simulink library "drives_lib"  (Simulink 6.0)
settings: Solver=ode45  SolverMode=SingleTasking  StartTime=0.0  StopTime=10.0  RelTol=1e-3
libraries: simulink_extras x2, simulink3 x1
settings Model: LastModifiedBy=studadm
settings OptimizationCC: BooleanDataType=off
settings DebuggingCC: SolverPrmCheckMsg=none
settings HardwareCC: TargetUnknown=on

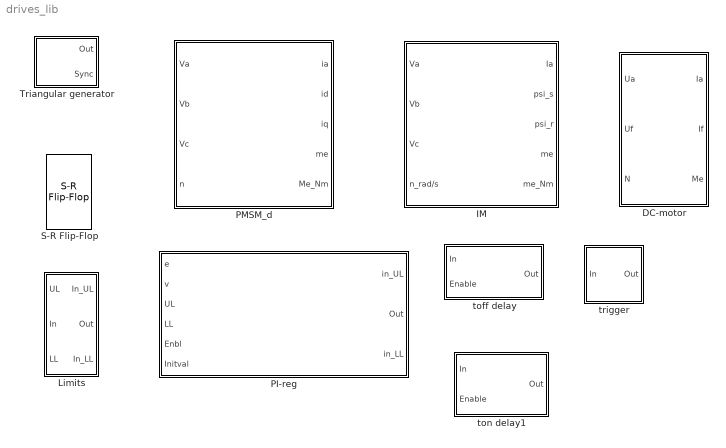
== system drives_lib ==
  DC-motor : Subsystem  mask{U_aN=400, I_aN=2.5, U_fN=310, I_fN=7, n_ref=1000, Ra_ref=160, MN=8, Ra=0.5, La=0.005, Tf=0.1}
      mask prompts: U_aN "U_an, anker merkespenning [V]"; I_aN "I_aN, anker merkestrøm [A]"; U_fN "U_fn, felt merkespenning [V]"; I_fN "I_fn, felt merkestrøm [A]"; n_ref "n_ref, merketurtall [o/min]"; Ra_ref "Ra_ref, basismotstand [ohm]"; MN "MN, merkemoment [Nm]"; Ra "Ra, ankermotstand [ohm]"; La "La, anker induktans [H]"; Tf "Tf, tidskonstant i feltkrets [sek]"
      mask help: DC-motor med skalering til pu-verdier
      mask Display:
      | text(0.25,0.7,'Likestrøm')
      | text(0.25,0.6,'maskin')
  IM : Subsystem  mask{Sn=10000, Un=400, fn=50, p=2, rs=0.04, rr=0.03, xh=2.273, xs=2.375, xr=2.385}
      mask prompts: Sn "Sn, merkeeffekt [VA]"; Un "Un, merke linjespenning [V]"; fn "fn, merkefrevens [Hz]"; p "p, antall polpar"; rs "rs, statorresistans [p.u]"; rr "rr, rotorresistans [p.u]"; xh "xh, magnetiseringsresistans [p.u]"; xs "xs, statorreaktans"; xr "xr, rotorreaktans"
      mask help:
      | Denne modulen er en asynkronmotormodul (kortslutningsmotor).
      | Modulen er basert paa invers-gamma transformasjonen.
      | Tilstandsvariable er stator strom i alfa og beta akse, og
      | rotor fluks i alfa og beta akse.
      mask Display:
      | text(0.20,0.9,'Induction machine')
      | 
      | 
      | plot([0.2500    0.2600    0.2700    0.2900    0.3100    0.3300    0.3600    0.3900    0.4200    0.4600    0.5000    0.5400    0.5800    0.6100    0.6400    0.6700    0.6900    0.7100    0.7300    0.7400    0.7500], [0.6000    0.6700    0.6980    0.7356    0.7625    0.7833    0.8071    0.8245    0.8369    0.8468    0.8500    0.8468    0.8369    0.8245    0.8071    0.7833    0.7625    0.7356    0.6980    0.6700    0.6000])
      | plot([0.2500    0.2600    0.2700    0.2900    0.3100    0.3300    0.3600    0.3900    0.4200    0.4600    0.5000    0.5400    0.5800    0.6100    0.6400    0.6700    0.6900    0.7100    0.7300    0.7400    0.7500], [0.6000    0.5300    0.5020    0.4644    0.4375    0.4167    0.3929    0.3755    0.3631    0.3532    0.3500    0.3532    0.3631    0.3755    0.3929    0.4167    0.4375    0.4644    0.5020    0.5300    0.6000])
      | 
      | plot([0.3250    0.3320    0.3390    0.3530    0.3670    0.3810    0.4020    0.4230    0.4440    0.4720    0.5000    0.5280    0.5560    0.5770    0.5980    0.6190    0.6330    0.6470    0.6610    0.6680    0.6750], [0.6000    0.6490    0.6686    0.6950    0.7137    0.7283    0.7450    0.7571    0.7658    0.7727    0.7750    0.7727    0.7658    0.7571    0.7450    0.7283    0.7137    0.6950    0.6686    0.6490    0.6000])
      | plot([0.3250    0.3320    0.3390    0.3530    0.3670    0.3810    0.4020    0.4230    0.4440    0.4720    0.5000    0.5280    0.5560    0.5770    0.5980    0.6190    0.6330    0.6470    0.6610    0.6680    0.6750], [0.6000    0.5510    0.5314    0.5050    0.4863    0.4717    0.4550    0.4429    0.4342    0.4273    0.4250    0.4273    0.4342    0.4429    0.4550    0.4717    0.4863    0.5050    0.5314    0.5510    0.6000])
      | 
      | plot([0.4 0.4 0.44 0.44 0.4],   [0.55 0.65 0.65 0.55 0.55])
      | plot([0.56 0.56 0.6 0.6 0.56], [0.55 0.65 0.65 0.55 0.55])
      | plot([0.45 0.55 0.55 0.45 0.45], [0.5 0.5 0.53 0.53 0.5])
      | plot([0.45 0.55 0.55 0.45 0.45], [0.7 0.7 0.67 0.67 0.7])
      | 
      | plot([0.495 0.505 0.755 0.745 0.495], [0.595 0.605 0.355 0.345 0.595])
  Limits : Subsystem
      mask Display:
      | plot([0.3 0.5 0.7 0.3], [0.1 0.3  0.1 0.1])
      | plot([0.3 0.5 0.7 0.3], [0.9 0.7  0.9 0.9])
  PI-reg : Subsystem  mask{Kp=0.3234, Kv=0, Ti=12e-3}
      mask Display:
      | plot([0.2 0.8], [0.1 0.1])
      | plot([0.2 0.2], [0.1 0.9])
      | plot([0.75 0.8 0.75], [0.15 0.1 0.05])
      | plot([0.175 0.2 0.225], [0.79 0.9 0.79])
      | 
      | plot([0.2 0.75], [0.3 0.7])
  PMSM_d : Subsystem  mask{Sn=3000, p=4, Un=230, fn=50, xd=0.5, xq=1.0, xls=0.06, xlkd=0.15, xlkq=0.15, rs=0.02, rkd=0.05, rkq=0.1, im=1.0}
      mask prompts: Sn "Sn, merkeeffekt [VA]"; p "p, antall polpar"; Un "Un, merkespenning (line-line rms) [V]"; fn "fn, merkefrekvens [Hz]"; xd "xd, reaktans i d-akse [p.u]"; xq "xq, reaktans i q-akse [p.u]"; xls "x_ls, lekkreaktans i stator [p.u]"; xlkd "x_lkd, lekkreaktans i dempevikl. d-akse [p.u]"; xlkq "x_lkq, lekkreaktans i dempevikl. q-akse [p.u]"; rs "rs, pr. fase statorresistans [p.u]"; rkd "r_kd, resistans i dempevikl. d-akse [p.u]"; rkq "r_kq, resistans i dempevikl. q-akse [p.u]"; im "i_m, ekv. magnetiseringsstrøm [p.u]"
      mask help:
      | dq-transformert modell av en permanentmagnetisert
      | synkronmotor (PMSM) med dempeviklinger.
      mask Display:
      | text(0.15,0.9,'PM Synch. Machine')
      | text(0.2,0.25,'w/damperwindings')
      | 
      | plot([0.2500    0.2600    0.2700    0.2900    0.3100    0.3300    0.3600    0.3900    0.4200    0.4600    0.5000    0.5400    0.5800    0.6100    0.6400    0.6700    0.6900    0.7100    0.7300    0.7400    0.7500], [0.6000    0.6700    0.6980    0.7356    0.7625    0.7833    0.8071    0.8245    0.8369    0.8468    0.8500    0.8468    0.8369    0.8245    0.8071    0.7833    0.7625    0.7356    0.6980    0.6700    0.6000])
      | plot([0.2500    0.2600    0.2700    0.2900    0.3100    0.3300    0.3600    0.3900    0.4200    0.4600    0.5000    0.5400    0.5800    0.6100    0.6400    0.6700    0.6900    0.7100    0.7300    0.7400    0.7500], [0.6000    0.5300    0.5020    0.4644    0.4375    0.4167    0.3929    0.3755    0.3631    0.3532    0.3500    0.3532    0.3631    0.3755    0.3929    0.4167    0.4375    0.4644    0.5020    0.5300    0.6000])
      | 
      | plot([0.3250    0.3320    0.3390    0.3530    0.3670    0.3810    0.4020    0.4230    0.4440    0.4720    0.5000    0.5280    0.5560    0.5770    0.5980    0.6190    0.6330    0.6470    0.6610    0.6680    0.6750], [0.6000    0.6490    0.6686    0.6950    0.7137    0.7283    0.7450    0.7571    0.7658    0.7727    0.7750    0.7727    0.7658    0.7571    0.7450    0.7283    0.7137    0.6950    0.6686    0.6490    0.6000])
      | plot([0.3250    0.3320    0.3390    0.3530    0.3670    0.3810    0.4020    0.4230    0.4440    0.4720    0.5000    0.5280    0.5560    0.5770    0.5980    0.6190    0.6330    0.6470    0.6610    0.6680    0.6750], [0.6000    0.5510    0.5314    0.5050    0.4863    0.4717    0.4550    0.4429    0.4342    0.4273    0.4250    0.4273    0.4342    0.4429    0.4550    0.4717    0.4863    0.5050    0.5314    0.5510    0.6000])
      | 
      | plot([0.4 0.4 0.44 0.44 0.4],   [0.55 0.65 0.65 0.55 0.55])
      | plot([0.56 0.56 0.6 0.6 0.56], [0.55 0.65 0.65 0.55 0.55])
      | plot([0.45 0.55 0.55 0.45 0.45], [0.5 0.5 0.53 0.53 0.5])
      | plot([0.45 0.55 0.55 0.45 0.45], [0.7 0.7 0.67 0.67 0.7])
      | 
      | plot([0.495 0.505 0.755 0.745 0.495], [0.595 0.605 0.355 0.345 0.595])
  S-R Flip-Flop : simulink_extras/Flip Flops/S-R Flip-Flop  initial_condition=0
  Triangular generator : Subsystem  mask(Triangular wave generator){ftri=1000, A=1, O=0}
      mask prompts: ftri "Frequency [Hz]"; A "Amplitude"; O "Offset"
      mask help:
      | Outputs a triangular waveform between -Amplitude and
      | +Amplitude with the set frequency and an optional offset.
      | The sync signal goes high at +Ampl. and low at -Ampl.
      mask Display: plot([0 0.1 0.2 0.3 0.4 0.5 0.6 ],[0 1 0 1 0 1 0])
  toff delay : Subsystem  mask{td=0.05}
      mask prompts: td "tidsforsinkelse td [s]:"
      mask help:
      | Når inngangen går høy, går utgangen momentant høy. Når inngangen går lav, går utgangen
      | lav etter en tidsforsinkelse td. Prosessen overstyres av Enable.
      mask Display:
      | plot([0.3 0.4 0.4 0.6 0.6 0.7 ],[0.7  0.7 1 1 0.7 0.7])
      | plot([0.3 0.4 0.4 0.65 0.65 0.7 ],[0.3  0.3 0.6 0.6 0.3 0.3])
  ton delay1 : Subsystem  AncestorBlock=eea_lib/ton delay  mask{td=0.8}
      mask prompts: td "tidsforsinkelse td [s]:"
      mask help:
      | Når inngangen går høy, går utgangen høy etter en tidsforsinkelse td. Når inngangen går lav, går utgangen
      | lavt momentant. Prosessen overstyres av Enable.
      mask Display:
      | plot([0.3 0.4 0.4 0.6 0.6 0.7 ],[0.7  0.7 1 1 0.7 0.7])
      | plot([0.3 0.45 0.45 0.6 0.6 0.7 ],[0.3  0.3 0.6 0.6 0.3 0.3])
  trigger : Subsystem  mask{ton=}
      mask prompts: ton "Påtid, ton [s]:"
      mask help:
      | Når inngangen går høy,
      |  går utgangen høy i en tid lik ton.
      mask Display:
      | plot([0.1 0.15 0.15 0.20 0.20 0.4  0.45 0.45 0.5 0.5 0.6],[0.7  0.7 1 1 0.7 0.7 0.7 1 1 0.7 0.7])
      | plot([0.1 0.15 0.15 0.35 0.35 0.4 0.45 0.45 0.6 ],[0.3 0.3 0.6 0.6 0.3 0.3 0.3 0.6 0.6])
      | plot([0.15 0.17],[0.48 0.48])
      | plot([0.33 0.35],[0.48 0.48])
      | text(0.21,0.5,'ton')

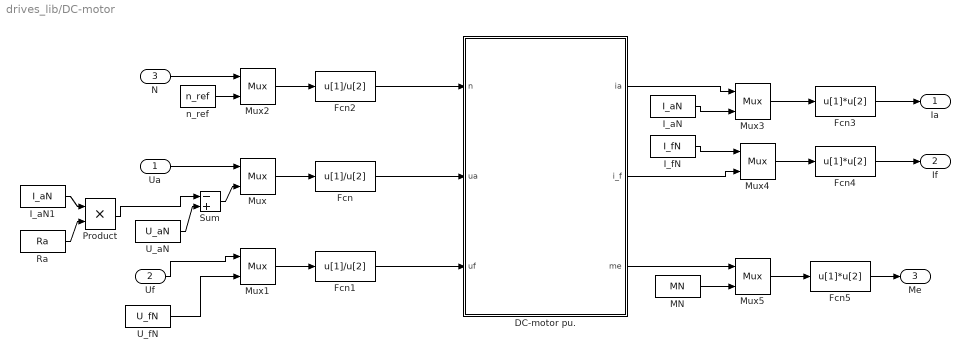
== system drives_lib/DC-motor ==
  Ua : Inport  Port=1  LatchInput=off
  Uf : Inport  Port=2  LatchInput=off
  N : Inport  Port=3  LatchInput=off
  DC-motor pu. : Subsystem
  Fcn : Fcn  Expr=u[1]/u[2]
  Fcn1 : Fcn  Expr=u[1]/u[2]
  Fcn2 : Fcn  Expr=u[1]/u[2]
  Fcn3 : Fcn  Expr=u[1]*u[2]
  Fcn4 : Fcn  Expr=u[1]*u[2]
  Fcn5 : Fcn  Expr=u[1]*u[2]
  I_aN : Constant  Value=I_aN
  I_aN1 : Constant  Value=I_aN
  I_fN : Constant  Value=I_fN
  MN : Constant  Value=MN
  Mux{,1..5} (6 alike) : Mux  Inputs=2
  Product : Product  SaturateOnIntegerOverflow=on  RndMeth=Zero  InputSameDT=on
  Ra : Constant  Value=Ra
  Sum : Sum  Inputs=-+  SaturateOnIntegerOverflow=on  InputSameDT=on
  U_aN : Constant  Value=U_aN
  U_fN : Constant  Value=U_fN
  n_ref : Constant  Value=n_ref
  Ia : Outport  InitialOutput=0
  If : Outport  Port=2  InitialOutput=0
  Me : Outport  Port=3  InitialOutput=0
  wires:
  N/1 -> Mux2/1
  Mux2/1 -> Fcn2/1
  n_ref/1 -> Mux2/2
  Fcn2/1 -> DC-motor pu./1(n)
  Ua/1 -> Mux/1
  Mux/1 -> Fcn/1
  Fcn/1 -> DC-motor pu./2(ua)
  Uf/1 -> Mux1/1
  Mux1/1 -> Fcn1/1
  Fcn1/1 -> DC-motor pu./3(uf)
  DC-motor pu./2(i_f) -> Mux4/2
  DC-motor pu./1(ia) -> Mux3/1
  I_aN/1 -> Mux3/2
  Mux3/1 -> Fcn3/1
  Mux4/1 -> Fcn4/1
  Fcn3/1 -> Ia/1
  Fcn4/1 -> If/1
  MN/1 -> Mux5/2
  Mux5/1 -> Fcn5/1
  Fcn5/1 -> Me/1
  DC-motor pu./3(me) -> Mux5/1
  Sum/1 -> Mux/2
  U_aN/1 -> Sum/2
  Product/1 -> Sum/1
  I_aN1/1 -> Product/1
  Ra/1 -> Product/2
  U_fN/1 -> Mux1/2
  I_fN/1 -> Mux4/1

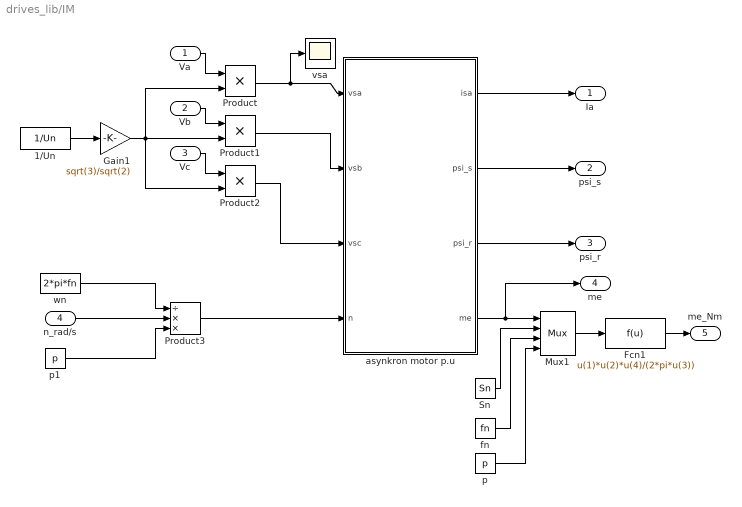
== system drives_lib/IM ==
  Va : Inport  Port=1  LatchInput=off
  Vb : Inport  Port=2  LatchInput=off
  Vc : Inport  Port=3  LatchInput=off
  n_rad/s : Inport  Port=4  LatchInput=off
  1/Un : Constant  Value=1/Un
  Fcn1 : Fcn  Expr=u(1)*u(2)*u(4)/(2*pi*u(3))
  Gain1 : Gain  Gain=sqrt(3)/sqrt(2)  SaturateOnIntegerOverflow=on
  Mux1 : Mux
  Product : Product  SaturateOnIntegerOverflow=on  RndMeth=Zero  InputSameDT=on
  Product1 : Product  SaturateOnIntegerOverflow=on  RndMeth=Zero  InputSameDT=on
  Product2 : Product  SaturateOnIntegerOverflow=on  RndMeth=Zero  InputSameDT=on
  Product3 : Product  Inputs=/**  SaturateOnIntegerOverflow=on  RndMeth=Zero  InputSameDT=on
  Sn : Constant  Value=Sn
  asynkron motor p.u : Subsystem
  fn : Constant  Value=fn
  p : Constant  Value=p
  p1 : Constant  Value=p
  vsa : Scope
      settings: TickLabels=on  YMin=-25  YMax=15  DataFormat=Array
  wn : Constant  Value=2*pi*fn
  Ia : Outport  InitialOutput=0
  psi_s : Outport  Port=2  InitialOutput=0
  psi_r : Outport  Port=3  InitialOutput=0
  me : Outport  Port=4  InitialOutput=0
  me_Nm : Outport  Port=5  InitialOutput=0
  wires:
  asynkron motor p.u/3(psi_r) -> psi_r/1
  asynkron motor p.u/2("psi_s ") -> psi_s/1
  Vc/1 -> Product2/1
  asynkron motor p.u/1(isa) -> Ia/1
  Vb/1 -> Product1/1
  Va/1 -> Product/1
  Product2/1 -> asynkron motor p.u/3(vsc)
  Product1/1 -> asynkron motor p.u/2(vsb)
  Fcn1/1 -> me_Nm/1
  Sn/1 -> Mux1/2
  Mux1/1 -> Fcn1/1
  fn/1 -> Mux1/3
  p/1 -> Mux1/4
  asynkron motor p.u/4(me) -> me/1, Mux1/1
  Gain1/1 -> Product1/2, Product/2, Product2/2
  1/Un/1 -> Gain1/1
  Product/1 -> asynkron motor p.u/1(vsa), vsa/1
  n_rad/s/1 -> Product3/2
  Product3/1 -> asynkron motor p.u/4(n)
  p1/1 -> Product3/3
  wn/1 -> Product3/1

== system drives_lib/Limits ==
  UL : Inport  Port=1  LatchInput=off
  In : Inport  Port=2  LatchInput=off
  LL : Inport  Port=3  LatchInput=off
  LL-test : MinMax  Function=max  Inputs=2  SaturateOnIntegerOverflow=on  InputSameDT=on
  Sum : Sum  Inputs=|-+  SaturateOnIntegerOverflow=on  InputSameDT=on
  Sum1 : Sum  Inputs=-+|  SaturateOnIntegerOverflow=on  InputSameDT=on
  UL-test : MinMax  Inputs=2  SaturateOnIntegerOverflow=on  InputSameDT=on
  in LL : Relay  OnSwitchValue=0  OffSwitchValue=-eps
  in UL : Relay  OnSwitchValue=0  OffSwitchValue=-eps
  In_UL : Outport
  Out : Outport  Port=2
  In_LL : Outport  Port=3
  wires:
  UL-test/1 -> LL-test/1, Sum/2
  Sum1/1 -> in LL/1
  LL-test/1 -> Sum1/1, Out/1
  UL/1 -> UL-test/1, Sum/1
  LL/1 -> LL-test/2, Sum1/2
  In/1 -> UL-test/2
  in LL/1 -> In_LL/1
  Sum/1 -> in UL/1
  in UL/1 -> In_UL/1

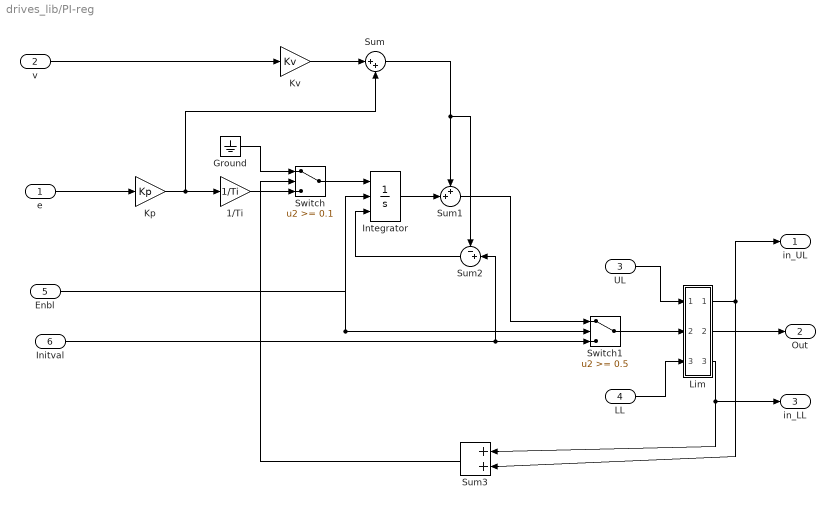
== system drives_lib/PI-reg ==
  e : Inport  Port=1  LatchInput=off
  v : Inport  Port=2  LatchInput=off
  UL : Inport  Port=3  LatchInput=off
  LL : Inport  Port=4  LatchInput=off
  Enbl : Inport  Port=5  LatchInput=off
  Initval : Inport  Port=6  LatchInput=off
  1/Ti : Gain  Gain=1/Ti  SaturateOnIntegerOverflow=on
  Ground : Ground
  Integrator : Integrator  ExternalReset=rising  InitialConditionSource=external
  Kp : Gain  Gain=Kp  SaturateOnIntegerOverflow=on
  Kv : Gain  Gain=Kv  SaturateOnIntegerOverflow=on
  Lim : Subsystem
      mask Display:
      | plot([0.3 0.5 0.7 0.3], [0.1 0.3  0.1 0.1])
      | plot([0.3 0.5 0.7 0.3], [0.9 0.7  0.9 0.9])
  Sum : Sum  Inputs=|++  SaturateOnIntegerOverflow=on  InputSameDT=on
  Sum1 : Sum  Inputs=++|  SaturateOnIntegerOverflow=on  InputSameDT=on
  Sum2 : Sum  Orientation=left  Inputs=-+|  SaturateOnIntegerOverflow=on  InputSameDT=on
  Sum3 : Sum  Orientation=left  Inputs=++|  SaturateOnIntegerOverflow=on  InputSameDT=on
  Switch : Switch  Threshold=0.1  SaturateOnIntegerOverflow=on  InputSameDT=on
  Switch1 : Switch  Threshold=0.5  SaturateOnIntegerOverflow=on  InputSameDT=on
  in_UL : Outport
  Out : Outport  Port=2
  in_LL : Outport  Port=3
  wires:
  Lim/3(In_LL) -> in_LL/1, Sum3/1
  Lim/2(Out) -> Out/1
  Lim/1(In_UL) -> in_UL/1, Sum3/2
  LL/1 -> Lim/3(LL)
  e/1 -> Kp/1
  UL/1 -> Lim/1(UL)
  v/1 -> Kv/1
  Sum3/1 -> Switch/2
  Sum2/1 -> Integrator/3
  Initval/1 -> Sum2/2, Switch1/3
  Sum/1 -> Sum2/1, Sum1/1
  Enbl/1 -> Integrator/2, Switch1/2
  Sum1/1 -> Switch1/1
  Integrator/1 -> Sum1/2
  Kp/1 -> Sum/2, 1/Ti/1
  Ground/1 -> Switch/1
  1/Ti/1 -> Switch/3
  Switch/1 -> Integrator/1
  Switch1/1 -> Lim/2(In)
  Kv/1 -> Sum/1

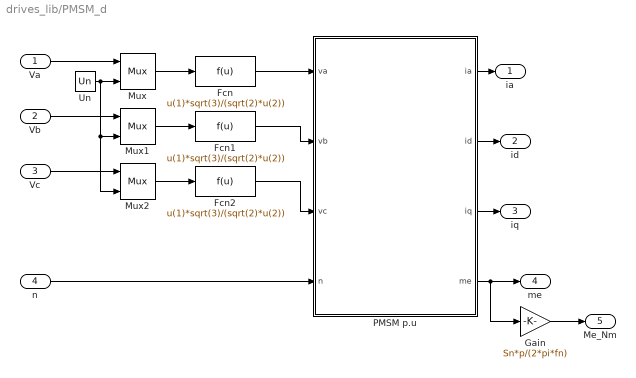
== system drives_lib/PMSM_d ==
  Va : Inport  Port=1  LatchInput=off
  Vb : Inport  Port=2  LatchInput=off
  Vc : Inport  Port=3  LatchInput=off
  n : Inport  Port=4  LatchInput=off
  Fcn : Fcn  Expr=u(1)*sqrt(3)/(sqrt(2)*u(2))
  Fcn1 : Fcn  Expr=u(1)*sqrt(3)/(sqrt(2)*u(2))
  Fcn2 : Fcn  Expr=u(1)*sqrt(3)/(sqrt(2)*u(2))
  Gain : Gain  Gain=Sn*p/(2*pi*fn)  SaturateOnIntegerOverflow=on
  Mux : Mux  Inputs=2
  Mux1 : Mux  Inputs=2
  Mux2 : Mux  Inputs=2
  PMSM p.u : Subsystem
  Un : Constant  Value=Un
  ia : Outport  InitialOutput=0
  id : Outport  Port=2  InitialOutput=0
  iq : Outport  Port=3  InitialOutput=0
  me : Outport  Port=4  InitialOutput=0
  Me_Nm : Outport  Port=5  InitialOutput=0
  wires:
  Mux/1 -> Fcn/1
  Fcn1/1 -> PMSM p.u/2(vb)
  Mux1/1 -> Fcn1/1
  Fcn2/1 -> PMSM p.u/3(vc)
  Mux2/1 -> Fcn2/1
  Un/1 -> Mux/2, Mux1/2, Mux2/2
  PMSM p.u/1(ia) -> ia/1
  PMSM p.u/2(id) -> id/1
  PMSM p.u/3(iq) -> iq/1
  Va/1 -> Mux/1
  Vb/1 -> Mux1/1
  Vc/1 -> Mux2/1
  n/1 -> PMSM p.u/4(n)
  Gain/1 -> Me_Nm/1
  PMSM p.u/4(me) -> me/1, Gain/1
  Fcn/1 -> PMSM p.u/1(va)

== system drives_lib/Triangular generator ==
  Constant : Constant  Value=O
  Constant1 : Constant  Value=A
  Fcn : Fcn  Expr=((u(1)-u(2))/(2*u(3)))+0.5
  Mux : Mux  Inputs=3
  Repeating Sequence : simulink3/Sources/Repeating Sequence  rep_seq_t=[0 1/(2*ftri) 1/ftri]  rep_seq_y="[-A  A  -A]"
  Sum : Sum  SaturateOnIntegerOverflow=on  InputSameDT=on
  Zero-Order Hold : ZeroOrderHold  SampleTime=1/(2*ftri)
  Out : Outport
  Sync : Outport  Port=2
  wires:
  Repeating Sequence/1 -> Sum/1
  Sum/1 -> Out/1, Zero-Order Hold/1
  Zero-Order Hold/1 -> Mux/1
  Mux/1 -> Fcn/1
  Fcn/1 -> Sync/1
  Constant/1 -> Sum/2, Mux/2
  Constant1/1 -> Mux/3

== system drives_lib/toff delay ==
  In : Inport  Port=1  LatchInput=off
  Enable : Inport  Port=2  LatchInput=off
  AND1 : Logic  Operator=OR
  AND2 : Logic
  Data Type Conversion : DataTypeConversion
  Data Type Conversion1 : DataTypeConversion
  Transport Delay1 : TransportDelay  DelayTime=td
  Out : Outport
  wires:
  In/1 -> AND1/1, Data Type Conversion1/1
  AND1/1 -> AND2/1
  AND2/1 -> Out/1
  Enable/1 -> AND2/2
  Data Type Conversion1/1 -> Transport Delay1/1
  Data Type Conversion/1 -> AND1/2
  Transport Delay1/1 -> Data Type Conversion/1

== system drives_lib/ton delay1 ==
  In : Inport  Port=1  LatchInput=off
  Enable : Inport  Port=2  LatchInput=off
  AND1 : Logic
  AND2 : Logic
  Data Type Conversion : DataTypeConversion
  Data Type Conversion1 : DataTypeConversion
  Transport Delay1 : TransportDelay  DelayTime=td
  Out : Outport
  wires:
  Enable/1 -> AND2/2
  AND2/1 -> Out/1
  AND1/1 -> AND2/1
  Data Type Conversion1/1 -> Transport Delay1/1
  In/1 -> AND1/1, Data Type Conversion1/1
  Data Type Conversion/1 -> AND1/2
  Transport Delay1/1 -> Data Type Conversion/1

== system drives_lib/trigger ==
  In : Inport  Port=1  LatchInput=off
  S-R Flip-Flop : simulink_extras/Flip Flops/S-R Flip-Flop  initial_condition=0
  Terminator : Terminator
  Transport Delay : TransportDelay  DelayTime=ton
  Out : Outport  Orientation=up
  wires:
  S-R Flip-Flop/2 -> Terminator/1
  S-R Flip-Flop/1 -> Transport Delay/1, Out/1
  Transport Delay/1 -> S-R Flip-Flop/2
  In/1 -> S-R Flip-Flop/1

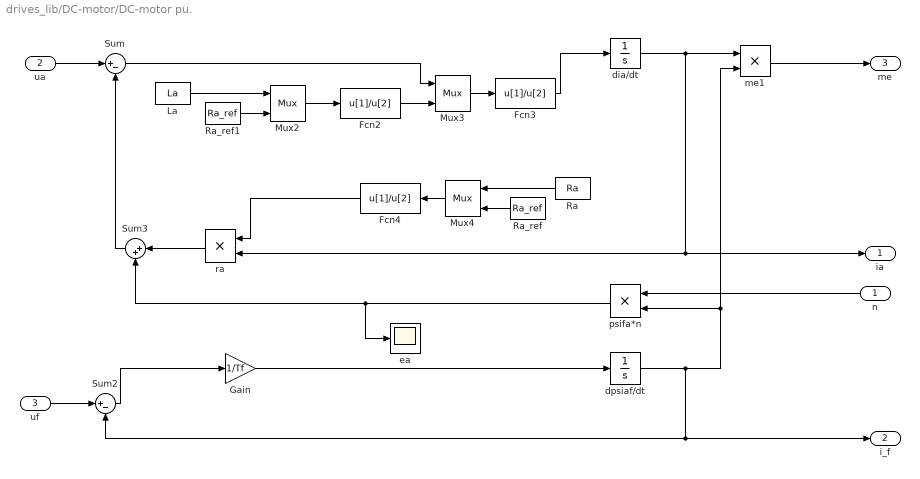
== system drives_lib/DC-motor/DC-motor pu. ==
  n : Inport  Orientation=left  Port=1  LatchInput=off
  ua : Inport  Port=2  LatchInput=off
  uf : Inport  Port=3  LatchInput=off
  Fcn2 : Fcn  Expr=u[1]/u[2]
  Fcn3 : Fcn  Expr=u[1]/u[2]
  Fcn4 : Fcn  Orientation=left  Expr=u[1]/u[2]
  Gain : Gain  Gain=1/Tf  SaturateOnIntegerOverflow=on
  La : Constant  Value=La
  Mux2 : Mux  Inputs=2
  Mux3 : Mux  Inputs=2
  Mux4 : Mux  Orientation=left  Inputs=2
  Ra : Constant  Orientation=left  Value=Ra
  Ra_ref : Constant  Orientation=left  Value=Ra_ref
  Ra_ref1 : Constant  Value=Ra_ref
  Sum : Sum  Inputs=|+-  SaturateOnIntegerOverflow=on  InputSameDT=on
  Sum2 : Sum  Inputs=|+-  SaturateOnIntegerOverflow=on  InputSameDT=on
  Sum3 : Sum  Orientation=left  Inputs=|++  SaturateOnIntegerOverflow=on  InputSameDT=on
  dia/dt : Integrator
  dpsiaf/dt : Integrator  LimitOutput=on  LowerSaturationLimit=0
  ea : Scope
      settings: YMin=0  YMax=2  DataFormat=Structure
  me1 : Product  SaturateOnIntegerOverflow=on  RndMeth=Zero  InputSameDT=on
  psifa*n : Product  Orientation=left  SaturateOnIntegerOverflow=on  RndMeth=Zero  InputSameDT=on
  ra : Product  Orientation=left  SaturateOnIntegerOverflow=on  RndMeth=Zero  InputSameDT=on
  ia : Outport
  i_f : Outport  Port=2
  me : Outport  Port=3
  wires:
  Sum3/1 -> Sum/2
  ua/1 -> Sum/1
  uf/1 -> Sum2/1
  me1/1 -> me/1
  dia/dt/1 -> me1/1, ia/1, ra/2
  La/1 -> Mux2/1
  Ra_ref1/1 -> Mux2/2
  Fcn2/1 -> Mux3/2
  Mux3/1 -> Fcn3/1
  dpsiaf/dt/1 -> me1/2, psifa*n/2, Sum2/2, i_f/1
  Gain/1 -> dpsiaf/dt/1
  n/1 -> psifa*n/1
  Fcn3/1 -> dia/dt/1
  Sum/1 -> Mux3/1
  Mux2/1 -> Fcn2/1
  Ra/1 -> Mux4/1
  Ra_ref/1 -> Mux4/2
  Mux4/1 -> Fcn4/1
  Sum2/1 -> Gain/1
  ra/1 -> Sum3/1
  Fcn4/1 -> ra/1
  psifa*n/1 -> Sum3/2, ea/1

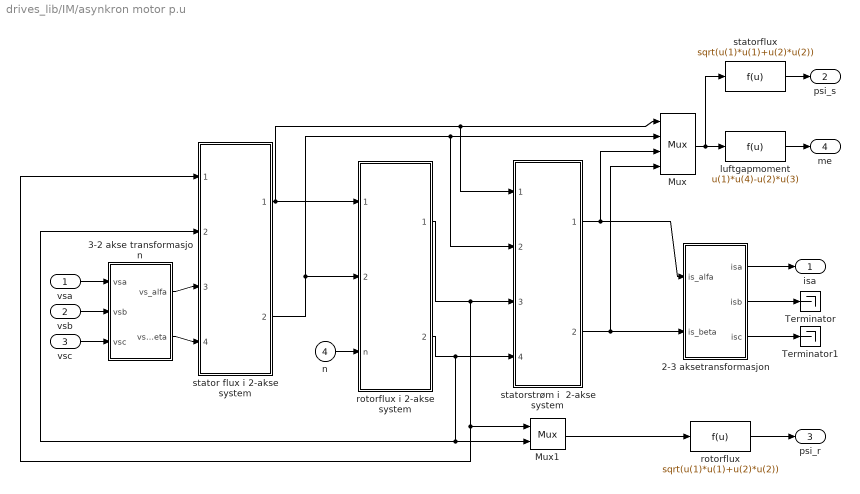
== system drives_lib/IM/asynkron motor p.u ==
  vsa : Inport  Port=1  LatchInput=off
  vsb : Inport  Port=2  LatchInput=off
  vsc : Inport  Port=3  LatchInput=off
  n : Inport  Port=4  LatchInput=off
  2-3 aksetransformasjon : Subsystem
  3-2 akse transformasjon : Subsystem
  Mux : Mux
  Mux1 : Mux  Inputs=2
  Terminator : Terminator
  Terminator1 : Terminator
  "luftgapmoment " : Fcn  Expr=u(1)*u(4)-u(2)*u(3)
  rotorflux : Fcn  Expr=sqrt(u(1)*u(1)+u(2)*u(2))
  rotorflux i 2-akse system : Subsystem
  stator flux i 2-akse system : Subsystem
  statorflux : Fcn  Expr=sqrt(u(1)*u(1)+u(2)*u(2))
  statorstrøm i  2-akse system : Subsystem
  isa : Outport  InitialOutput=0
  "psi_s " : Outport  Port=2  InitialOutput=0
  psi_r : Outport  Port=3  InitialOutput=0
  me : Outport  Port=4  InitialOutput=0
  wires:
  2-3 aksetransformasjon/1(isa) -> isa/1
  "luftgapmoment "/1 -> me/1
  statorstrøm i  2-akse system/1(is_alfa) -> Mux/3, 2-3 aksetransformasjon/1(is_alfa)
  statorstrøm i  2-akse system/2(is_beta) -> Mux/4, 2-3 aksetransformasjon/2(is_beta)
  n/1 -> rotorflux i 2-akse system/3(n)
  stator flux i 2-akse system/1(psis_alfa) -> rotorflux i 2-akse system/1(psis_alfa), statorstrøm i  2-akse system/1(psis_alfa), Mux/1
  stator flux i 2-akse system/2(psis_beta) -> rotorflux i 2-akse system/2(psis_beta), statorstrøm i  2-akse system/2(psis_beta), Mux/2
  vsa/1 -> 3-2 akse transformasjon/1(vsa)
  vsb/1 -> 3-2 akse transformasjon/2(vsb)
  vsc/1 -> 3-2 akse transformasjon/3(vsc)
  3-2 akse transformasjon/1(vs_alfa) -> stator flux i 2-akse system/3(vs_alfa)
  3-2 akse transformasjon/2(vs_beta) -> stator flux i 2-akse system/4(vs_beta)
  rotorflux i 2-akse system/2(psir_beta) -> statorstrøm i  2-akse system/4(psir_beta), stator flux i 2-akse system/2(psir_beta), Mux1/2
  rotorflux i 2-akse system/1(psir_alfa) -> statorstrøm i  2-akse system/3(psir_alfa), stator flux i 2-akse system/1(psir_alfa), Mux1/1
  Mux/1 -> "luftgapmoment "/1, statorflux/1
  2-3 aksetransformasjon/2(isb) -> Terminator/1
  2-3 aksetransformasjon/3(isc) -> Terminator1/1
  statorflux/1 -> "psi_s "/1
  rotorflux/1 -> psi_r/1
  Mux1/1 -> rotorflux/1

== system drives_lib/PI-reg/Lim ==
  UL : Inport  Port=1  LatchInput=off
  In : Inport  Port=2  LatchInput=off
  LL : Inport  Port=3  LatchInput=off
  LL-test : MinMax  Function=max  Inputs=2  SaturateOnIntegerOverflow=on  InputSameDT=on
  Sum : Sum  Inputs=|-+  SaturateOnIntegerOverflow=on  InputSameDT=on
  Sum1 : Sum  Inputs=-+|  SaturateOnIntegerOverflow=on  InputSameDT=on
  UL-test : MinMax  Inputs=2  SaturateOnIntegerOverflow=on  InputSameDT=on
  in LL : Relay  OnSwitchValue=0  OffSwitchValue=-eps
  in UL : Relay  OnSwitchValue=0  OffSwitchValue=-eps
  In_UL : Outport
  Out : Outport  Port=2
  In_LL : Outport  Port=3
  wires:
  in UL/1 -> In_UL/1
  Sum/1 -> in UL/1
  in LL/1 -> In_LL/1
  In/1 -> UL-test/2
  LL/1 -> Sum1/2, LL-test/2
  UL/1 -> Sum/1, UL-test/1
  LL-test/1 -> Out/1, Sum1/1
  Sum1/1 -> in LL/1
  UL-test/1 -> Sum/2, LL-test/1

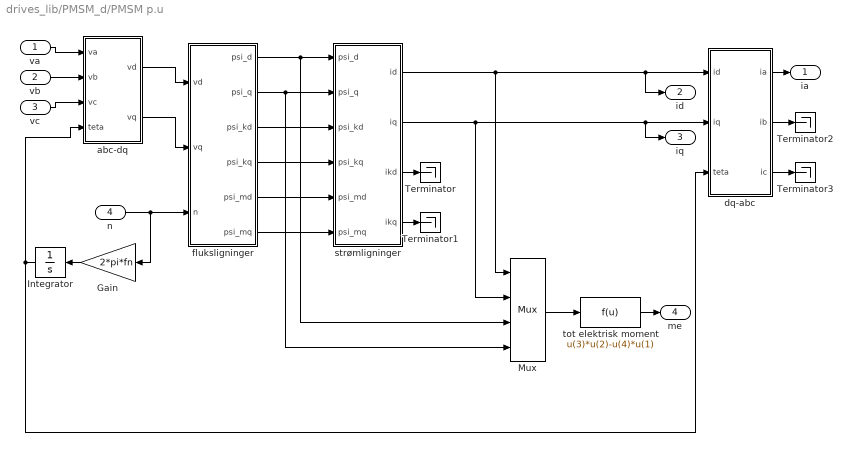
== system drives_lib/PMSM_d/PMSM p.u ==
  va : Inport  Port=1  LatchInput=off
  vb : Inport  Port=2  LatchInput=off
  vc : Inport  Port=3  LatchInput=off
  n : Inport  Port=4  LatchInput=off
  Gain : Gain  Orientation=left  Gain=2*pi*fn  SaturateOnIntegerOverflow=on
  Integrator : Integrator  Orientation=left
  Mux : Mux
  Terminator{,1..3} (4 alike) : Terminator
  abc-dq : Subsystem
  dq-abc : Subsystem
  fluksligninger : Subsystem
  strømligninger : Subsystem
  tot elektrisk moment : Fcn  Expr=u(3)*u(2)-u(4)*u(1)
  ia : Outport  InitialOutput=0
  id : Outport  Port=2  InitialOutput=0
  iq : Outport  Port=3  InitialOutput=0
  me : Outport  Port=4  InitialOutput=0
  wires:
  va/1 -> abc-dq/1(va)
  abc-dq/1(vd) -> fluksligninger/1(vd)
  abc-dq/2(vq) -> fluksligninger/2(vq)
  vb/1 -> abc-dq/2(vb)
  vc/1 -> abc-dq/3(vc)
  fluksligninger/3(psi_kd) -> strømligninger/3(psi_kd)
  fluksligninger/4(psi_kq) -> strømligninger/4(psi_kq)
  fluksligninger/6(psi_mq) -> strømligninger/6(psi_mq)
  n/1 -> fluksligninger/3(n), Gain/1
  Gain/1 -> Integrator/1
  Integrator/1 -> abc-dq/4(teta), dq-abc/3(teta)
  tot elektrisk moment/1 -> me/1
  strømligninger/3(ikd) -> Terminator/1
  strømligninger/4(ikq) -> Terminator1/1
  fluksligninger/5(psi_md) -> strømligninger/5(psi_md)
  dq-abc/1(ia) -> ia/1
  fluksligninger/1(psi_d) -> strømligninger/1(psi_d), Mux/3
  fluksligninger/2("psi_q ") -> strømligninger/2(psi_q), Mux/4
  strømligninger/1(id) -> Mux/1, dq-abc/1(id), id/1
  strømligninger/2(iq) -> Mux/2, dq-abc/2(iq), iq/1
  dq-abc/2(ib) -> Terminator2/1
  dq-abc/3(ic) -> Terminator3/1
  Mux/1 -> tot elektrisk moment/1

== system drives_lib/IM/asynkron motor p.u/2-3 aksetransformasjon ==
  is_alfa : Inport  Port=1  LatchInput=off
  is_beta : Inport  Port=2  LatchInput=off
  Fcn : Fcn  Expr=-0.5*u(1)+sqrt(3)*u(2)/2
  Fcn1 : Fcn  Expr=-0.5*u(1)-sqrt(3)*u(2)/2
  Mux : Mux  Inputs=2
  isa : Outport  InitialOutput=0
  isb : Outport  Port=2  InitialOutput=0
  isc : Outport  Port=3  InitialOutput=0
  wires:
  is_beta/1 -> Mux/2
  is_alfa/1 -> Mux/1, isa/1
  Fcn/1 -> isb/1
  Fcn1/1 -> isc/1
  Mux/1 -> Fcn/1, Fcn1/1

== system drives_lib/IM/asynkron motor p.u/3-2 akse transformasjon ==
  note: 3 til 2 aksetransformasjon
  vsa : Inport  Port=1  LatchInput=off
  vsb : Inport  Port=2  LatchInput=off
  vsc : Inport  Port=3  LatchInput=off
  Fcn : Fcn  Expr=(u(1)-u(2))/sqrt(3)
  Mux : Mux  Inputs=2
  vs_alfa : Outport  InitialOutput=0
  vs_beta : Outport  Port=2  InitialOutput=0
  wires:
  vsc/1 -> Mux/2
  vsb/1 -> Mux/1
  Mux/1 -> Fcn/1
  Fcn/1 -> vs_beta/1
  vsa/1 -> vs_alfa/1

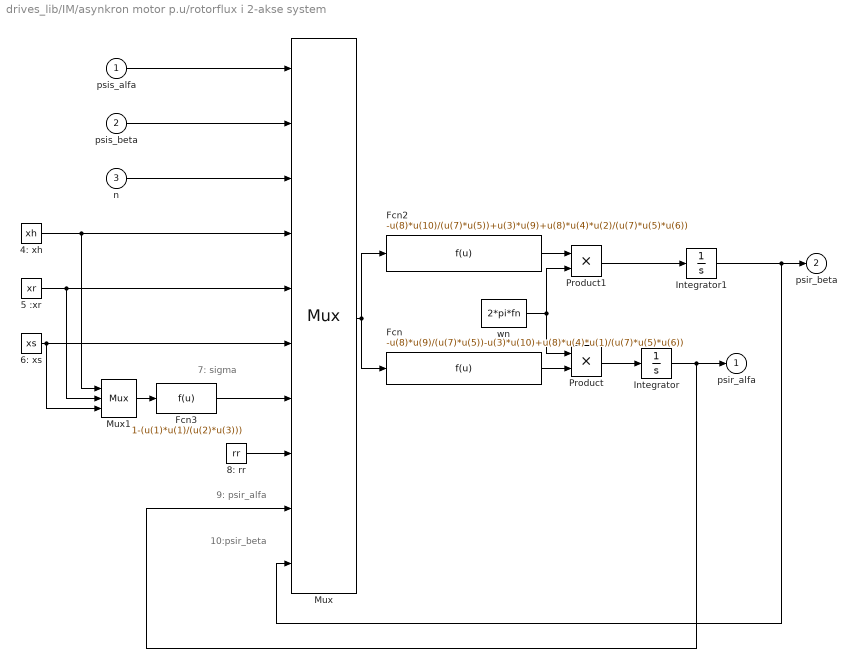
== system drives_lib/IM/asynkron motor p.u/rotorflux i 2-akse system ==
  note: 9: psir_alfa
  note: 10:psir_beta
  note: 7: sigma
  psis_alfa : Inport  Port=1  LatchInput=off
  psis_beta : Inport  Port=2  LatchInput=off
  n : Inport  Port=3  LatchInput=off
  4: xh : Constant  Value=xh
  5 :xr : Constant  Value=xr
  6: xs : Constant  Value=xs
  8: rr : Constant  Value=rr
  Fcn : Fcn  Expr=-u(8)*u(9)/(u(7)*u(5))-u(3)*u(10)+u(8)*u(4)*u(1)/(u(7)*u(5)*u(6))
  Fcn2 : Fcn  Expr=-u(8)*u(10)/(u(7)*u(5))+u(3)*u(9)+u(8)*u(4)*u(2)/(u(7)*u(5)*u(6))
  Fcn3 : Fcn  Expr=1-(u(1)*u(1)/(u(2)*u(3)))
  Integrator : Integrator
  Integrator1 : Integrator
  Mux : Mux  Inputs=10
  Mux1 : Mux  Inputs=3
  Product : Product  SaturateOnIntegerOverflow=on  RndMeth=Zero  InputSameDT=on
  Product1 : Product  SaturateOnIntegerOverflow=on  RndMeth=Zero  InputSameDT=on
  wn : Constant  Value=2*pi*fn
  psir_alfa : Outport  InitialOutput=0
  psir_beta : Outport  Port=2  InitialOutput=0
  wires:
  Product/1 -> Integrator/1
  Mux/1 -> Fcn/1, Fcn2/1
  Fcn2/1 -> Product1/1
  Product1/1 -> Integrator1/1
  psis_alfa/1 -> Mux/1
  psis_beta/1 -> Mux/2
  n/1 -> Mux/3
  wn/1 -> Product1/2, Product/1
  Fcn/1 -> Product/2
  Mux1/1 -> Fcn3/1
  4: xh/1 -> Mux1/1, Mux/4
  5 :xr/1 -> Mux1/2, Mux/5
  6: xs/1 -> Mux1/3, Mux/6
  8: rr/1 -> Mux/8
  Integrator/1 -> psir_alfa/1, Mux/9
  Integrator1/1 -> psir_beta/1, Mux/10
  Fcn3/1 -> Mux/7

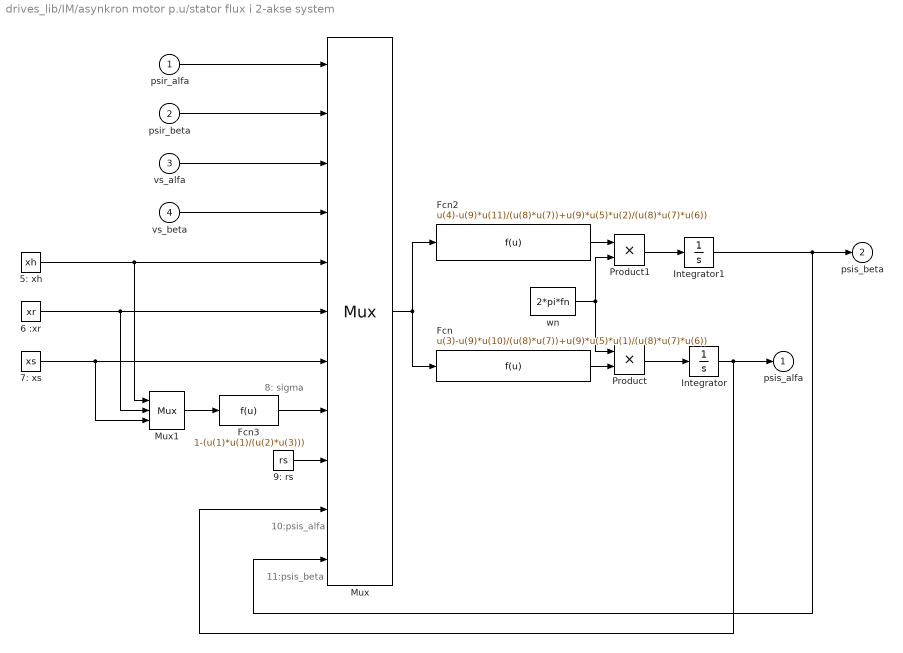
== system drives_lib/IM/asynkron motor p.u/stator flux i 2-akse system ==
  note: 10:psis_alfa
  note: 11:psis_beta
  note: 8: sigma
  psir_alfa : Inport  Port=1  LatchInput=off
  psir_beta : Inport  Port=2  LatchInput=off
  vs_alfa : Inport  Port=3  LatchInput=off
  vs_beta : Inport  Port=4  LatchInput=off
  5: xh : Constant  Value=xh
  6 :xr : Constant  Value=xr
  7: xs : Constant  Value=xs
  9: rs : Constant  Value=rs
  Fcn : Fcn  Expr=u(3)-u(9)*u(10)/(u(8)*u(7))+u(9)*u(5)*u(1)/(u(8)*u(7)*u(6))
  Fcn2 : Fcn  Expr=u(4)-u(9)*u(11)/(u(8)*u(7))+u(9)*u(5)*u(2)/(u(8)*u(7)*u(6))
  Fcn3 : Fcn  Expr=1-(u(1)*u(1)/(u(2)*u(3)))
  Integrator : Integrator
  Integrator1 : Integrator
  Mux : Mux  Inputs=11
  Mux1 : Mux  Inputs=3
  Product : Product  SaturateOnIntegerOverflow=on  RndMeth=Zero  InputSameDT=on
  Product1 : Product  SaturateOnIntegerOverflow=on  RndMeth=Zero  InputSameDT=on
  wn : Constant  Value=2*pi*fn
  psis_alfa : Outport  InitialOutput=0
  psis_beta : Outport  Port=2  InitialOutput=0
  wires:
  Product/1 -> Integrator/1
  Mux/1 -> Fcn/1, Fcn2/1
  Fcn2/1 -> Product1/1
  Product1/1 -> Integrator1/1
  psir_alfa/1 -> Mux/1
  psir_beta/1 -> Mux/2
  vs_alfa/1 -> Mux/3
  wn/1 -> Product1/2, Product/1
  Fcn/1 -> Product/2
  Mux1/1 -> Fcn3/1
  vs_beta/1 -> Mux/4
  5: xh/1 -> Mux1/1, Mux/5
  6 :xr/1 -> Mux1/2, Mux/6
  7: xs/1 -> Mux1/3, Mux/7
  Fcn3/1 -> Mux/8
  9: rs/1 -> Mux/9
  Integrator/1 -> psis_alfa/1, Mux/10
  Integrator1/1 -> psis_beta/1, Mux/11

== system drives_lib/IM/asynkron motor p.u/statorstrøm i  2-akse system ==
  psis_alfa : Inport  Port=1  LatchInput=off
  psis_beta : Inport  Port=2  LatchInput=off
  psir_alfa : Inport  Port=3  LatchInput=off
  psir_beta : Inport  Port=4  LatchInput=off
  5: xs : Constant  Value=xs
  6: xh : Constant  Value=xh
  7: xr : Constant  Value=xr
  Fcn : Fcn  Expr=(u(7)*u(2)-u(6)*u(4))/(u(5)*u(7)-u(6)*u(6))
  Fcn1 : Fcn  Expr=(u(7)*u(1)-u(6)*u(3))/(u(5)*u(7)-u(6)*u(6))
  Mux : Mux  Inputs=7
  is_alfa : Outport  InitialOutput=0
  is_beta : Outport  Port=2  InitialOutput=0
  wires:
  psis_beta/1 -> Mux/2
  psis_alfa/1 -> Mux/1
  psir_alfa/1 -> Mux/3
  psir_beta/1 -> Mux/4
  5: xs/1 -> Mux/5
  6: xh/1 -> Mux/6
  Fcn1/1 -> is_alfa/1
  Fcn/1 -> is_beta/1
  7: xr/1 -> Mux/7
  Mux/1 -> Fcn/1, Fcn1/1

== system drives_lib/PMSM_d/PMSM p.u/abc-dq ==
  va : Inport  Port=1  LatchInput=off
  vb : Inport  Port=2  LatchInput=off
  vc : Inport  Port=3  LatchInput=off
  teta : Inport  Port=4  LatchInput=off
  Fcn : Fcn  Expr=2*(u(1)*cos(u(4))+u(2)*cos(u(4)-2*pi/3)+u(3)*cos(u(4)+2*pi/3))/3
  Fcn1 : Fcn  Expr=2*(-u(1)*sin(u(4))-u(2)*sin(u(4)-2*pi/3)-u(3)*sin(u(4)+2*pi/3))/3
  Mux : Mux
  vd : Outport  InitialOutput=0
  vq : Outport  Port=2  InitialOutput=0
  wires:
  Mux/1 -> Fcn/1, Fcn1/1
  Fcn/1 -> vd/1
  va/1 -> Mux/1
  vb/1 -> Mux/2
  vc/1 -> Mux/3
  teta/1 -> Mux/4
  Fcn1/1 -> vq/1

== system drives_lib/PMSM_d/PMSM p.u/dq-abc ==
  id : Inport  Port=1  LatchInput=off
  iq : Inport  Port=2  LatchInput=off
  teta : Inport  Port=3  LatchInput=off
  Fcn : Fcn  Expr=u(1)*cos(u(3))-u(2)*sin(u(3))
  Fcn1 : Fcn  Expr=u(1)*cos(u(3)-2*pi/3)-u(2)*sin(u(3)-2*pi/3)
  Fcn2 : Fcn  Expr=u(1)*cos(u(3)+2*pi/3)-u(2)*sin(u(3)+2*pi/3)
  Mux : Mux  Inputs=3
  ia : Outport  InitialOutput=0
  ib : Outport  Port=2  InitialOutput=0
  ic : Outport  Port=3  InitialOutput=0
  wires:
  Mux/1 -> Fcn/1, Fcn1/1, Fcn2/1
  Fcn/1 -> ia/1
  id/1 -> Mux/1
  iq/1 -> Mux/2
  teta/1 -> Mux/3
  Fcn1/1 -> ib/1
  Fcn2/1 -> ic/1

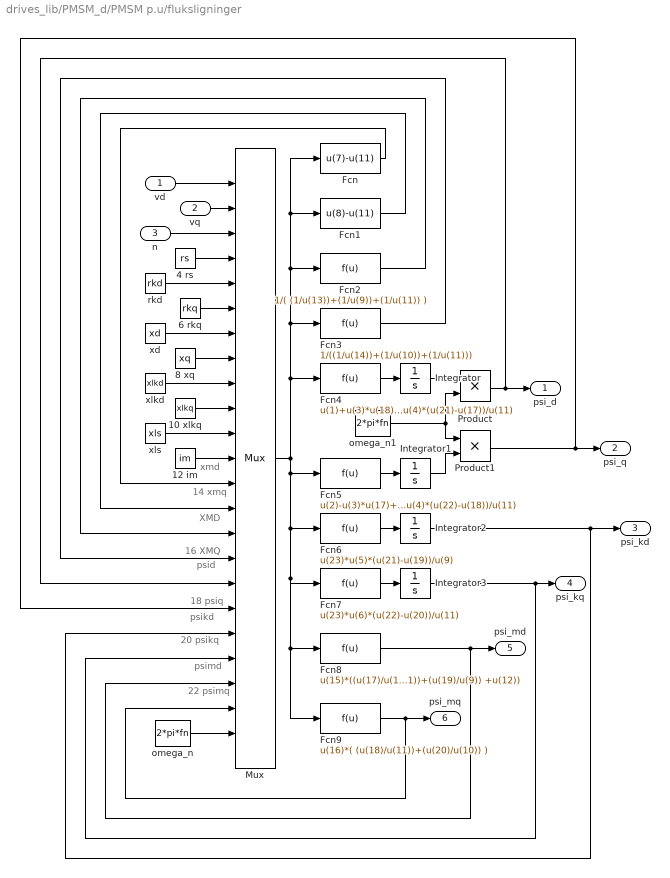
== system drives_lib/PMSM_d/PMSM p.u/fluksligninger ==
  note: xmd
  note: 14 xmq
  note: XMD
  note: 16 XMQ
  note: psid
  note: 18 psiq
  note: psikd
  note: 20 psikq
  note: psimd
  note: 22 psimq
  vd : Inport  Port=1  LatchInput=off
  vq : Inport  Port=2  LatchInput=off
  n : Inport  Port=3  LatchInput=off
  "  xlkd" : Constant  Value=xlkd
  "  xls" : Constant  Value=xls
  " rkd" : Constant  Value=rkd
  " xd" : Constant  Value=xd
  10 xlkq : Constant  Value=xlkq
  12 im : Constant  Value=im
  4 rs : Constant  Value=rs
  6 rkq : Constant  Value=rkq
  8 xq : Constant  Value=xq
  Fcn : Fcn  Expr=u(7)-u(11)
  Fcn1 : Fcn  Expr=u(8)-u(11)
  Fcn2 : Fcn  Expr=1/( (1/u(13))+(1/u(9))+(1/u(11)) )
  Fcn3 : Fcn  Expr=1/((1/u(14))+(1/u(10))+(1/u(11)))
  Fcn4 : Fcn  Expr=u(1)+u(3)*u(18)+u(4)*(u(21)-u(17))/u(11)
  Fcn5 : Fcn  Expr=u(2)-u(3)*u(17)+u(4)*(u(22)-u(18))/u(11)
  Fcn6 : Fcn  Expr=u(23)*u(5)*(u(21)-u(19))/u(9)
  Fcn7 : Fcn  Expr=u(23)*u(6)*(u(22)-u(20))/u(11)
  Fcn8 : Fcn  Expr=u(15)*((u(17)/u(11))+(u(19)/u(9)) +u(12))
  Fcn9 : Fcn  Expr=u(16)*( (u(18)/u(11))+(u(20)/u(10)) )
  Integrator{,1..3} (4 alike) : Integrator
  Mux : Mux  Inputs=23
  Product : Product  SaturateOnIntegerOverflow=on  RndMeth=Zero  InputSameDT=on
  Product1 : Product  SaturateOnIntegerOverflow=on  RndMeth=Zero  InputSameDT=on
  omega_n : Constant  Value=2*pi*fn
  omega_n1 : Constant  Value=2*pi*fn
  psi_d : Outport  InitialOutput=0
  "psi_q " : Outport  Port=2  InitialOutput=0
  psi_kd : Outport  Port=3  InitialOutput=0
  psi_kq : Outport  Port=4  InitialOutput=0
  psi_md : Outport  Port=5  InitialOutput=0
  psi_mq : Outport  Port=6  InitialOutput=0
  wires:
  Fcn/1 -> Mux/13
  Fcn1/1 -> Mux/14
  Fcn2/1 -> Mux/15
  Fcn3/1 -> Mux/16
  vd/1 -> Mux/1
  vq/1 -> Mux/2
  omega_n/1 -> Mux/23
  Fcn4/1 -> Integrator/1
  Mux/1 -> Fcn/1, Fcn1/1, Fcn2/1, Fcn3/1, Fcn4/1, Fcn5/1, Fcn6/1, Fcn7/1, Fcn8/1, Fcn9/1
  Integrator/1 -> Product/1
  Product/1 -> psi_d/1, Mux/17
  omega_n1/1 -> Product/2, Product1/1
  Fcn5/1 -> Integrator1/1
  Integrator1/1 -> Product1/2
  Product1/1 -> "psi_q "/1, Mux/18
  Fcn6/1 -> Integrator2/1
  Fcn7/1 -> Integrator3/1
  Fcn9/1 -> psi_mq/1, Mux/22
  Fcn8/1 -> psi_md/1, Mux/21
  Integrator3/1 -> psi_kq/1, Mux/20
  Integrator2/1 -> psi_kd/1, Mux/19
  n/1 -> Mux/3
  4 rs/1 -> Mux/4
  12 im/1 -> Mux/12
  " rkd"/1 -> Mux/5
  6 rkq/1 -> Mux/6
  " xd"/1 -> Mux/7
  8 xq/1 -> Mux/8
  "  xlkd"/1 -> Mux/9
  10 xlkq/1 -> Mux/10
  "  xls"/1 -> Mux/11

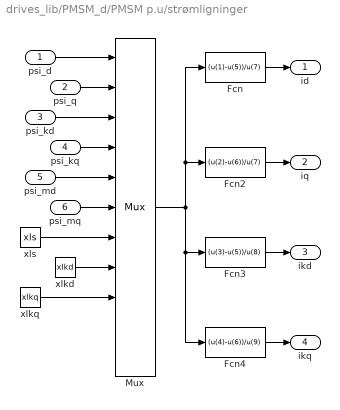
== system drives_lib/PMSM_d/PMSM p.u/strømligninger ==
  psi_d : Inport  Port=1  LatchInput=off
  psi_q : Inport  Port=2  LatchInput=off
  psi_kd : Inport  Port=3  LatchInput=off
  psi_kq : Inport  Port=4  LatchInput=off
  psi_md : Inport  Port=5  LatchInput=off
  psi_mq : Inport  Port=6  LatchInput=off
  Fcn : Fcn  Expr=(u(1)-u(5))/u(7)
  Fcn2 : Fcn  Expr=(u(2)-u(6))/u(7)
  Fcn3 : Fcn  Expr=(u(3)-u(5))/u(8)
  Fcn4 : Fcn  Expr=(u(4)-u(6))/u(9)
  Mux : Mux  Inputs=11
  xlkd : Constant  Value=xlkd
  xlkq : Constant  Value=xlkq
  xls : Constant  Value=xls
  id : Outport  InitialOutput=0
  iq : Outport  Port=2  InitialOutput=0
  ikd : Outport  Port=3  InitialOutput=0
  ikq : Outport  Port=4  InitialOutput=0
  wires:
  psi_d/1 -> Mux/1
  psi_q/1 -> Mux/2
  psi_kd/1 -> Mux/3
  psi_kq/1 -> Mux/4
  psi_md/1 -> Mux/5
  psi_mq/1 -> Mux/6
  xls/1 -> Mux/7
  xlkd/1 -> Mux/8
  xlkq/1 -> Mux/9
  Fcn/1 -> id/1
  Fcn2/1 -> iq/1
  Mux/1 -> Fcn/1, Fcn2/1, Fcn3/1, Fcn4/1
  Fcn3/1 -> ikd/1
  Fcn4/1 -> ikq/1
